simulink model "Control_System_Framework"  (R2024b)
settings: Solver=VariableStepAuto  StartTime=0.0  StopTime=10.0  RelTol=1e-3
settings Model: Creator=PME406_01  LastModifiedBy=kevin

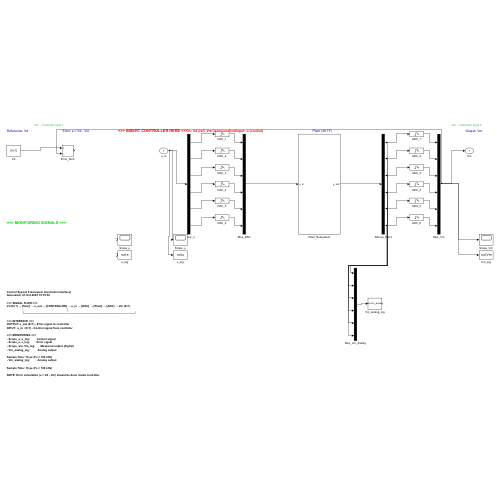
[thumbnail: Simulink's stored preview of the top-level diagram]
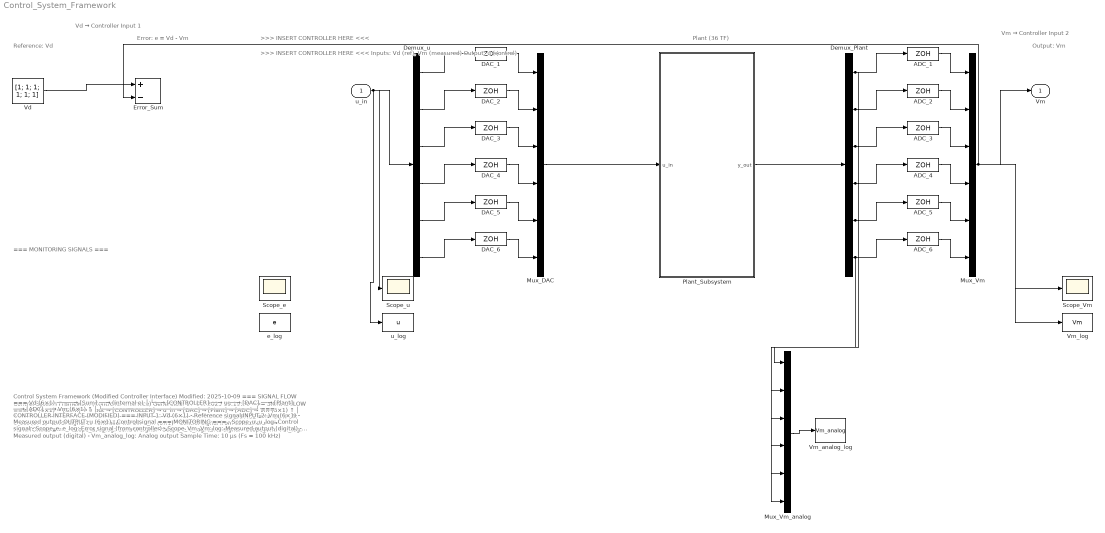
== system Control_System_Framework ==
  note: Control System Framework (Controller Interface)
      | Generated: 07-Oct-2025 19:19:30
      |
      | === SIGNAL FLOW ===
      | Vd (6×1) → [Sum] → e_out → [CONTROLLER] → u_in → [DAC] → [Plant] → [ADC] → Vm (6×1)
      |                     ↑                                                        │
      |                     └────────────────────────────────────────────────────────┘
      |
      | === INTERFACE ===
      | OUTPUT: e_out (6×1) - Error signal to controller
      | INPUT:  u_in  (6×1) - Control signal from controller
      |
      | === MONITORING ===
      | - Scope_u, u_log:         Control signal
      | - Scope_e, e_log:         Error signal
      | - Scope_Vm, Vm_log:       Measured output (digital)
      | - Vm_analog_log:          Analog output
      |
      | Sample Time: 10 μs (Fs = 100 kHz)
  note: Reference: Vd
  note: Error: e = Vd - Vm
  note: >>> INSERT CONTROLLER HERE <<<
  note: Plant (36 TF)
  note: Output: Vm
  note: === MONITORING SIGNALS ===
  note: Vd → Controller Input 1
  note: Vm → Controller Input 2
  note: >>> INSERT CONTROLLER HERE <<<\nInputs: Vd (ref), Vm (measured)\nOutput: u (control)
  note: Control System Framework (Modified Controller Interface)
      | Modified: 2025-10-09
      |
      | === SIGNAL FLOW ===
      | Vd (6×1) ──┬──→ [Sum] ──→ (internal e)
      |            │
      |            └──→ [CONTROLLER] ──→ u ──→ [DAC] ──→ [Plant] ──→ [ADC] ──→ Vm (6×1)
      |                      ↑                                              │
      |                      └──────────────────────────────────────────────┘
      |
      | === CONTROLLER INTERFACE (MODIFIED) ===
      | INPUT 1:  Vd (6×1) - Reference signal
      | INPUT 2:  Vm (6×1) - Measured output
      | OUTPUT:   u  (6×1) - Control signal
      |
      | === MONITORING ===
      | - Scope_u, u_log:         Control signal
      | - Scope_e, e_log:         Error signal (from controller)
      | - Scope_Vm, Vm_log:       Measured output (digital)
      | - Vm_analog_log:          Analog output
      |
      | Sample Time: 10 μs (Fs = 100 kHz)
      |
      | NOTE: Error calculation (e = Vd - Vm) should be done inside controller
  u_in : Inport
  ADC_{1..6} (6 alike) : ZeroOrderHold  SampleTime=1e-05
  DAC_{1..6} (6 alike) : ZeroOrderHold  SampleTime=1e-05
  Demux_Plant : Demux  Outputs=6
  Demux_u : Demux  Outputs=6
  Error_Sum : Sum  Inputs=+-
  Mux_DAC : Mux  Inputs=6
  Mux_Vm : Mux  Inputs=6
  Mux_Vm_analog : Mux  Inputs=6
  Plant_Subsystem : Subsystem
  Scope_Vm : Scope
  Scope_e : Scope
  Scope_u : Scope
  Vd : Constant  Value=[1; 1; 1; 1; 1; 1]  SampleTime=1e-05
  Vm_analog_log : ToWorkspace  VariableName=Vm_analog  SaveFormat=Timeseries  SampleTime=-1
  Vm_log : ToWorkspace  VariableName=Vm  SaveFormat=Timeseries  SampleTime=-1
  e_log : ToWorkspace  VariableName=e  SaveFormat=Timeseries  SampleTime=-1
  u_log : ToWorkspace  VariableName=u  SaveFormat=Timeseries  SampleTime=-1
  Vm : Outport
  wires:
  Vd/1 -> Error_Sum/1
  u_in/1 -> Demux_u/1, Scope_u/1, u_log/1
  Demux_u/1 -> DAC_1/1
  Demux_u/2 -> DAC_2/1
  Demux_u/3 -> DAC_3/1
  Demux_u/4 -> DAC_4/1
  Demux_u/5 -> DAC_5/1
  Demux_u/6 -> DAC_6/1
  DAC_1/1 -> Mux_DAC/1
  DAC_2/1 -> Mux_DAC/2
  DAC_3/1 -> Mux_DAC/3
  DAC_4/1 -> Mux_DAC/4
  DAC_5/1 -> Mux_DAC/5
  DAC_6/1 -> Mux_DAC/6
  Mux_DAC/1 -> Plant_Subsystem/1(u_in)
  Plant_Subsystem/1(y_out) -> Demux_Plant/1
  Demux_Plant/1 -> ADC_1/1, Mux_Vm_analog/1
  Demux_Plant/2 -> ADC_2/1, Mux_Vm_analog/2
  Demux_Plant/3 -> ADC_3/1, Mux_Vm_analog/3
  Demux_Plant/4 -> ADC_4/1, Mux_Vm_analog/4
  Demux_Plant/5 -> ADC_5/1, Mux_Vm_analog/5
  Demux_Plant/6 -> ADC_6/1, Mux_Vm_analog/6
  ADC_1/1 -> Mux_Vm/1
  ADC_2/1 -> Mux_Vm/2
  ADC_3/1 -> Mux_Vm/3
  ADC_4/1 -> Mux_Vm/4
  ADC_5/1 -> Mux_Vm/5
  ADC_6/1 -> Mux_Vm/6
  Mux_Vm/1 -> Vm/1, Error_Sum/2, Scope_Vm/1, Vm_log/1
  Mux_Vm_analog/1 -> Vm_analog_log/1

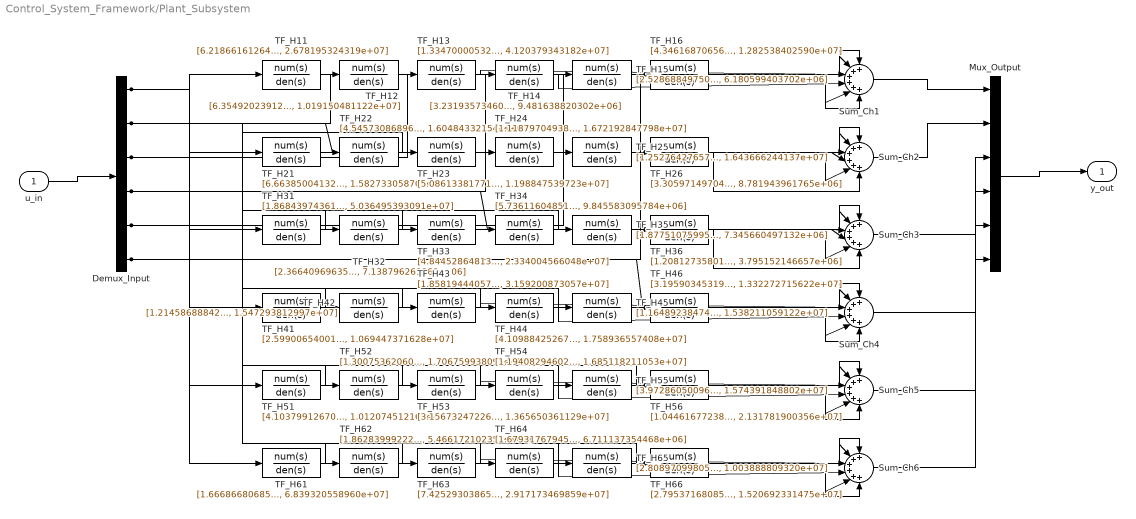
== system Control_System_Framework/Plant_Subsystem ==
  u_in : Inport
  Demux_Input : Demux  Outputs=6
  Mux_Output : Mux  Inputs=6
  Sum_Ch{1..6} (6 alike) : Sum  Inputs=++++++
  TF_H11 : TransferFcn  Numerator=[6.218661612646e+06]  Denominator=[1, 1.338651505722e+04, 2.678195324319e+07]
  TF_H12 : TransferFcn  Numerator=[6.354920239120e+04]  Denominator=[1, 1.662975234098e+03, 1.019150481122e+07]
  TF_H13 : TransferFcn  Numerator=[1.334700005324e+06]  Denominator=[1, 1.275258720887e+04, 4.120379343182e+07]
  TF_H14 : TransferFcn  Numerator=[3.231935734603e+05]  Denominator=[1, 7.852044258687e+03, 9.481638820302e+06]
  TF_H15 : TransferFcn  Numerator=[2.528688497505e+05]  Denominator=[1, 5.879364609866e+03, 6.180599403702e+06]
  TF_H16 : TransferFcn  Numerator=[4.346168706564e+05]  Denominator=[1, 3.929701077901e+03, 1.282538402590e+07]
  TF_H21 : TransferFcn  Numerator=[6.663850041322e+04]  Denominator=[1, 1.462325866359e+03, 1.582733058702e+07]
  TF_H22 : TransferFcn  Numerator=[4.545730868967e+06]  Denominator=[1, 1.062107240072e+04, 1.604843321544e+07]
  TF_H23 : TransferFcn  Numerator=[5.086133817713e+05]  Denominator=[1, 8.903580767443e+03, 1.198847539723e+07]
  TF_H24 : TransferFcn  Numerator=[1.118797049382e+06]  Denominator=[1, 1.187110606946e+04, 1.672192847798e+07]
  TF_H25 : TransferFcn  Numerator=[1.252764276578e+06]  Denominator=[1, 1.157065537065e+04, 1.643666244137e+07]
  TF_H26 : TransferFcn  Numerator=[3.305971497046e+05]  Denominator=[1, 7.320553639319e+03, 8.781943961765e+06]
  TF_H31 : TransferFcn  Numerator=[1.868439743615e+06]  Denominator=[1, 2.001759478912e+04, 5.036495393091e+07]
  TF_H32 : TransferFcn  Numerator=[2.366409696351e+05]  Denominator=[1, 5.555556272703e+03, 7.138796269860e+06]
  TF_H33 : TransferFcn  Numerator=[4.844528648136e+06]  Denominator=[1, 9.879529061686e+03, 2.334004566048e+07]
  TF_H34 : TransferFcn  Numerator=[5.736116048513e+04]  Denominator=[1, 1.969312774925e+03, 9.845583095784e+06]
  TF_H35 : TransferFcn  Numerator=[1.877510759958e+05]  Denominator=[1, 5.415723666298e+03, 7.345660497132e+06]
  TF_H36 : TransferFcn  Numerator=[1.208127358015e+05]  Denominator=[1, 1.223159436233e+03, 3.795152146657e+06]
  TF_H41 : TransferFcn  Numerator=[2.599006540014e+05]  Denominator=[1, 7.067011596941e+03, 1.069447371628e+07]
  TF_H42 : TransferFcn  Numerator=[1.214586888427e+06]  Denominator=[1, 1.068737062822e+04, 1.547293812997e+07]
  TF_H43 : TransferFcn  Numerator=[1.858194440575e+05]  Denominator=[1, 3.263628987101e+03, 3.159200873057e+07]
  TF_H44 : TransferFcn  Numerator=[4.109884252673e+06]  Denominator=[1, 1.197023152306e+04, 1.758936557408e+07]
  TF_H45 : TransferFcn  Numerator=[1.164892384743e+06]  Denominator=[1, 1.147497418550e+04, 1.538211059122e+07]
  TF_H46 : TransferFcn  Numerator=[3.195903453190e+05]  Denominator=[1, 8.115803419255e+03, 1.332272715622e+07]
  TF_H51 : TransferFcn  Numerator=[4.103799126701e+05]  Denominator=[1, 8.911718423988e+03, 1.012074512169e+07]
  TF_H52 : TransferFcn  Numerator=[1.300753620602e+06]  Denominator=[1, 1.129883111396e+04, 1.706759938095e+07]
  TF_H53 : TransferFcn  Numerator=[3.156732472269e+05]  Denominator=[1, 7.923123695230e+03, 1.365650361129e+07]
  TF_H54 : TransferFcn  Numerator=[1.194082946029e+06]  Denominator=[1, 1.165860639982e+04, 1.685118211053e+07]
  TF_H55 : TransferFcn  Numerator=[3.972860500964e+06]  Denominator=[1, 1.114673978611e+04, 1.574391848802e+07]
  TF_H56 : TransferFcn  Numerator=[1.044616772387e+05]  Denominator=[1, 1.795313113853e+03, 2.131781900356e+07]
  TF_H61 : TransferFcn  Numerator=[1.666866806856e+06]  Denominator=[1, 2.393920383335e+04, 6.839320558960e+07]
  TF_H62 : TransferFcn  Numerator=[1.862839992228e+05]  Denominator=[1, 4.466579568847e+03, 5.466172102353e+06]
  TF_H63 : TransferFcn  Numerator=[7.425293038651e+05]  Denominator=[1, 9.585044147566e+03, 2.917173469859e+07]
  TF_H64 : TransferFcn  Numerator=[1.679317679458e+05]  Denominator=[1, 5.027625797834e+03, 6.711137354468e+06]
  TF_H65 : TransferFcn  Numerator=[2.808970998056e+04]  Denominator=[1, 4.816641149236e+02, 1.003888809320e+07]
  TF_H66 : TransferFcn  Numerator=[2.795371680855e+06]  Denominator=[1, 6.650113581422e+03, 1.520692331475e+07]
  y_out : Outport
  wires:
  u_in/1 -> Demux_Input/1
  Demux_Input/1 -> TF_H11/1, TF_H21/1, TF_H31/1, TF_H41/1, TF_H51/1, TF_H61/1
  TF_H11/1 -> Sum_Ch1/1
  Demux_Input/2 -> TF_H12/1, TF_H22/1, TF_H32/1, TF_H42/1, TF_H52/1, TF_H62/1
  TF_H12/1 -> Sum_Ch1/2
  Demux_Input/3 -> TF_H13/1, TF_H23/1, TF_H33/1, TF_H43/1, TF_H53/1, TF_H63/1
  TF_H13/1 -> Sum_Ch1/3
  Demux_Input/4 -> TF_H14/1, TF_H24/1, TF_H34/1, TF_H44/1, TF_H54/1, TF_H64/1
  TF_H14/1 -> Sum_Ch1/4
  Demux_Input/5 -> TF_H15/1, TF_H25/1, TF_H35/1, TF_H45/1, TF_H55/1, TF_H65/1
  TF_H15/1 -> Sum_Ch1/5
  Demux_Input/6 -> TF_H16/1, TF_H26/1, TF_H36/1, TF_H46/1, TF_H56/1, TF_H66/1
  TF_H16/1 -> Sum_Ch1/6
  TF_H21/1 -> Sum_Ch2/1
  TF_H22/1 -> Sum_Ch2/2
  TF_H23/1 -> Sum_Ch2/3
  TF_H24/1 -> Sum_Ch2/4
  TF_H25/1 -> Sum_Ch2/5
  TF_H26/1 -> Sum_Ch2/6
  TF_H31/1 -> Sum_Ch3/1
  TF_H32/1 -> Sum_Ch3/2
  TF_H33/1 -> Sum_Ch3/3
  TF_H34/1 -> Sum_Ch3/4
  TF_H35/1 -> Sum_Ch3/5
  TF_H36/1 -> Sum_Ch3/6
  TF_H41/1 -> Sum_Ch4/1
  TF_H42/1 -> Sum_Ch4/2
  TF_H43/1 -> Sum_Ch4/3
  TF_H44/1 -> Sum_Ch4/4
  TF_H45/1 -> Sum_Ch4/5
  TF_H46/1 -> Sum_Ch4/6
  TF_H51/1 -> Sum_Ch5/1
  TF_H52/1 -> Sum_Ch5/2
  TF_H53/1 -> Sum_Ch5/3
  TF_H54/1 -> Sum_Ch5/4
  TF_H55/1 -> Sum_Ch5/5
  TF_H56/1 -> Sum_Ch5/6
  TF_H61/1 -> Sum_Ch6/1
  TF_H62/1 -> Sum_Ch6/2
  TF_H63/1 -> Sum_Ch6/3
  TF_H64/1 -> Sum_Ch6/4
  TF_H65/1 -> Sum_Ch6/5
  TF_H66/1 -> Sum_Ch6/6
  Sum_Ch1/1 -> Mux_Output/1
  Sum_Ch2/1 -> Mux_Output/2
  Sum_Ch3/1 -> Mux_Output/3
  Sum_Ch4/1 -> Mux_Output/4
  Sum_Ch5/1 -> Mux_Output/5
  Sum_Ch6/1 -> Mux_Output/6
  Mux_Output/1 -> y_out/1
